simulink model "cm_ssb"  (R2015b)
settings: Solver=ode45  StartTime=0.0  StopTime=10.0  RelTol=1e-3
undefined symbols (not defined in the file or in its folder): commblksprivate, Info
libraries: commanapbnd3 x2
settings Model: ExtModeAutoUpdateStatusClock=off  Creator=The MathWorks, Inc.  LastModifiedBy=Shravankumar147
settings DataIOCC: SaveFormat=Array  SignalLoggingName=logsOut
settings OptimizationCC: BlockReduction=off  BooleanDataType=off  ExpressionDepthLimit=2147483647  InitFltsAndDblsToZero=on
settings DebuggingCC: SaveWithParameterizedLinksMsg=none  UnderspecifiedInitializationDetection=Classic  MergeDetectMultiDrivingBlocksExec=none  SignalResolutionControl=TryResolveAllWithWarning  MultiTaskDSMMsg=warning  MultiTaskCondExecSysMsg=none  FcnCallInpInsideContextMsg=UseLocalSettings  StateNameClashWarn=warning
settings HardwareCC: ProdBitPerPointer=32  ProdLargestAtomicFloat=None  ProdIntDivRoundTo=Undefined  ProdEndianess=Unspecified  ProdWordSize=32  ProdHWDeviceType=Specified
settings CodeAppCC: MangleLength=5
settings GRTTargetCC: TargetFcnLib=ansi_tfl_tmw.mat  GeneratePreprocessorConditionals=Disable all  CombineOutputUpdateFcns=off  GRTInterface=on
settings ConfigComp: CovModelRefEnable=Off

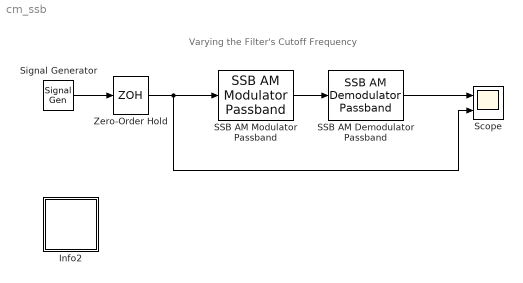
== system cm_ssb ==
  note: Varying the Filter's Cutoff Frequency
  Info2 : Subsystem  AncestorBlock=commblksprivate/Info  mask(Info){}
      settings: OpenFcn=helpview([docroot '/toolbox/comm/comm.map'], 'doc_filtercutoffs')
      mask Display: disp('Info')
  SSB AM Demodulator Passband : commanapbnd3/SSB AM Demodulator Passband  Fc=25  Ph=0  method=Butterworth  n=2  cf=30  Rp=0.1  Rs=50
  SSB AM Modulator Passband : commanapbnd3/SSB AM Modulator Passband  Fc=25  Ph=0  Sd=Upper  Ho=200
  Scope : Scope  NumInputPorts=2
  Signal Generator : SignalGenerator  WaveForm=sawtooth  Amplitude=4  Frequency=.3
  Zero-Order Hold : ZeroOrderHold  SampleTime=.01
  wires:
  Signal Generator/1 -> Zero-Order Hold/1
  SSB AM Modulator Passband/1 -> SSB AM Demodulator Passband/1
  SSB AM Demodulator Passband/1 -> Scope/1
  Zero-Order Hold/1 -> SSB AM Modulator Passband/1, Scope/2

== system cm_ssb/Info2 ==
